simulink model "Studio7b"  (R2017b)
settings: Solver=ode45  StartTime=0.  StopTime=60  MaxStep=0.05  RelTol=1e-8  AbsTol=1e-8  EnableMultiTasking=on
settings Model: ExtModeTrigMode=oneshot  ExtModeArmWhenConnect=off  Creator=LEVIENKL  LastModifiedBy=carlislt
settings DataIOCC: SaveFormat=Array  SignalLoggingSaveFormat=ModelDataLogs  SaveOutput=off  SaveTime=off  SignalLoggingName=sigsOut
settings OptimizationCC: BlockReduction=off  BooleanDataType=off  ExpressionDepthLimit=2147483647  InitFltsAndDblsToZero=on  LifeSpan=inf
settings DebuggingCC: SaveWithParameterizedLinksMsg=none  UnderspecifiedInitializationDetection=Classic  MergeDetectMultiDrivingBlocksExec=none  SignalResolutionControl=TryResolveAllWithWarning  MultiTaskDSMMsg=warning  MultiTaskCondExecSysMsg=none  FcnCallInpInsideContextMsg=warning  AllowSymbolicDim=off  StateNameClashWarn=warning  SFUnexpectedBacktrackingDiag=warning  SFNoUnconditionalDefaultTransitionDiag=warning  SFExecutionAtInitializationDiag=none
settings HardwareCC: ProdBitPerPointer=32  ProdBitPerSizeT=32  ProdBitPerPtrDiffT=32  ProdLargestAtomicFloat=None  ProdIntDivRoundTo=Undefined  ProdEndianess=Unspecified  ProdWordSize=32  ProdHWDeviceType=32-bit Generic  TargetUnknown=on
settings ModelReferenceCC: PropagateSignalLabelsOutOfModel=off
settings CodeAppCC: StateflowObjectComments=on
settings GRTTargetCC: TargetFcnLib=ansi_tfl_tmw.mat  TargetLangStandard=C89/C90 (ANSI)  GeneratePreprocessorConditionals=Disable all  CombineOutputUpdateFcns=off  GRTInterface=on
settings ConfigComp: CovMetricSettings=dw  CovHtmlReporting=on  CovSaveCumulativeToWorkspaceVar=on  CovSaveSingleToWorkspaceVar=on  CovExternalEMLEnable=off  CovSFcnEnable=off

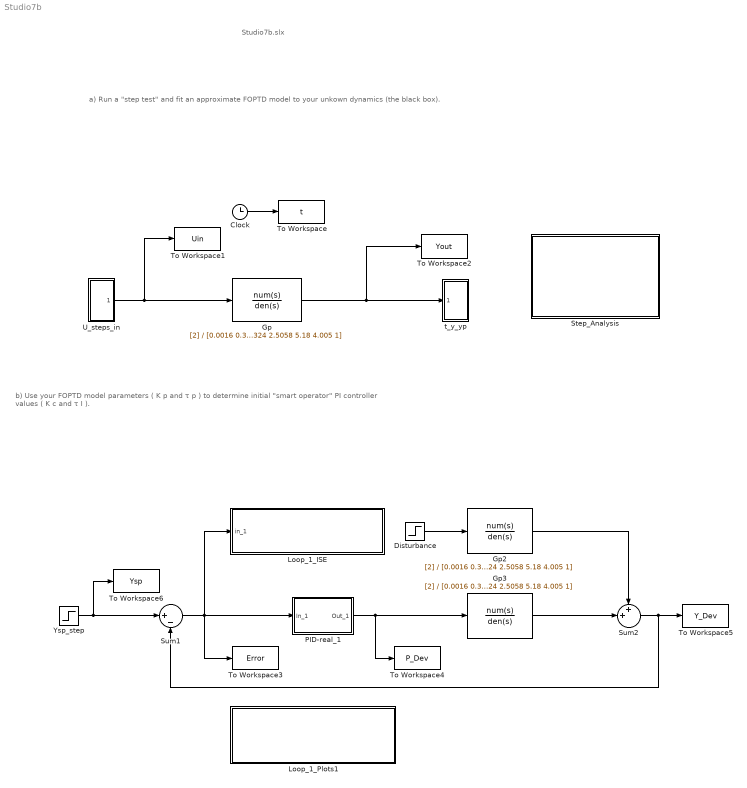
== system Studio7b ==
  note: Studio7b.slx
  note: a) Run a "step test" and fit an approximate FOPTD model to your unkown dynamics (the black box).
  note: b) Use your FOPTD model parameters ( K p and τ p ) to determine initial "smart operator" PI controller values ( K c and τ I ).
  Clock : Clock
  Disturbance : Step  Time=5  After=0  SampleTime=0
      settings: AttributesFormatString=%<Before> to %<After>\nat %<Time>
  Gp : TransferFcn  Numerator=[2]  Denominator=[0.0016 0.3324 2.5058 5.18 4.005 1]
  Gp2 : TransferFcn  Numerator=[2]  Denominator=[0.0016 0.3324 2.5058 5.18 4.005 1]
  Gp3 : TransferFcn  Numerator=[2]  Denominator=[0.0016 0.3324 2.5058 5.18 4.005 1]
  Loop_1_ISE : Subsystem  mask(Integral Squarred Evaluation - Loop 1){}
      settings: OpenFcn=ISE1
      mask Help: This block calculates and plots loop #1 ISE.
      mask Display: disp('After Loop 1 Simulation:\n Double Click for ISE evaluation\n (uses ISE1.p)')
  Loop_1_Plots1 : Subsystem  mask(Y,U,E Plots - Loop 1){}
      settings: OpenFcn=YPEplots
      mask Help: This block loop #1 Y,U,Error in 3x1 Figure Window.
      mask Display: disp('After Loop 1 Simulation:\n Double Click for Y, P, Error Plots\n (uses YPEplots.p)')
  PID-real_1 : Subsystem  mask(PID(with alpha) Controller for ChE 461){Kc=0.1, tauIi=1/10, tauD=0, alpha=0.05}
      mask prompts: Kc "Controller gain:"; tauIi "Inv of Integral time constant (careful - this is I action ! ) :"; tauD "Derivative time constant:"; alpha "Alpha value (small)::"
      mask help:
      | Enter expressions for controller gain,
      | inverse of integral time constant
      | and derivative time constant and alpha.
      settings: AttributesFormatString=Kc = %<Kc>\n1/TauI = %<tauIi>\nTauD = %<tauD>
      mask Help: This block implements a PID controller where parameters are entered for the Controller Gain, inverse of Integral time constant and Derivative time constant.  Alpha here is equal to 0.01.   Unmask this block to see how it works. The derivative term is implemented using a true derivative block.
      mask Display: disp('PIDalpha')
  Step_Analysis : Subsystem  mask(ASCII Datafile){}
      settings: OpenFcn=save tuin.dat tUin -ascii; save tyout.dat tYout -ascii; step2g
      mask Help: This block runs step2g\nin the MATLAB Command Window\nwith latest yout.dat data file.
      mask Display: disp('DOUBLE Click to\nRUN step2g\n\nGO TO Command Window !!')
  Sum1 : Sum  Inputs=|+-  SaturateOnIntegerOverflow=on  InputSameDT=on  OutDataTypeStr=Inherit: Same as first input
  Sum2 : Sum  Inputs=++|  SaturateOnIntegerOverflow=on  InputSameDT=on  OutDataTypeStr=Inherit: Same as first input
  To Workspace : ToWorkspace  VariableName=t  SampleTime=-1
  To Workspace1 : ToWorkspace  VariableName=Uin  SampleTime=-1
  To Workspace2 : ToWorkspace  VariableName=Yout  SampleTime=-1
  To Workspace3 : ToWorkspace  VariableName=Error  SampleTime=-1
  To Workspace4 : ToWorkspace  VariableName=P_Dev  SampleTime=-1
  To Workspace5 : ToWorkspace  VariableName=Y_Dev  SampleTime=-1
  To Workspace6 : ToWorkspace  VariableName=Ysp  SampleTime=-1
  U_steps_in : Subsystem
  Ysp_step : Step  Time=5  SampleTime=0
      settings: AttributesFormatString=%<Before> to %<After>\nat %<Time>
  t_y_yp : Subsystem
  wires:
  U_steps_in/1(out_1) -> To Workspace1/1, Gp/1
  Clock/1 -> To Workspace/1
  Gp/1 -> To Workspace2/1, t_y_yp/1(in_1)
  Disturbance/1 -> Gp2/1
  Gp3/1 -> Sum2/2
  PID-real_1/1(Out_1) -> Gp3/1, To Workspace4/1
  Gp2/1 -> Sum2/1
  Sum2/1 -> Sum1/2, To Workspace5/1
  Ysp_step/1 -> Sum1/1, To Workspace6/1
  Sum1/1 -> To Workspace3/1, Loop_1_ISE/1(in_1), PID-real_1/1(In_1)

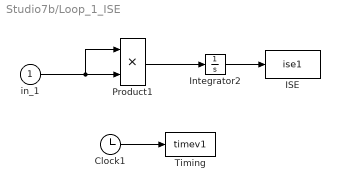
== system Studio7b/Loop_1_ISE ==
  in_1 : Inport
  Clock1 : Clock
  ISE : ToWorkspace  VariableName=ise1
      settings: MaxDataPoints=20000
  Integrator2 : Integrator
  Product1 : Product  SaturateOnIntegerOverflow=on  RndMeth=Zero  InputSameDT=on  OutDataTypeStr=Inherit: Same as first input
  Timing : ToWorkspace  VariableName=timev1
      settings: MaxDataPoints=20000
  wires:
  in_1/1 -> Product1/2, Product1/1
  Integrator2/1 -> ISE/1
  Clock1/1 -> Timing/1
  Product1/1 -> Integrator2/1

== system Studio7b/Loop_1_Plots1 ==

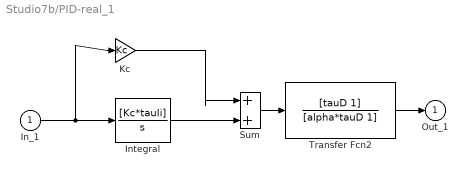
== system Studio7b/PID-real_1 ==
  In_1 : Inport
  Integral : TransferFcn  Numerator=[Kc*tauIi]  Denominator=[1 0]
  Kc : Gain  Gain=Kc  SaturateOnIntegerOverflow=on  OutDataTypeStr=Inherit: Same as input  ParamDataTypeStr=Inherit: Same as input
  Sum : Sum  SaturateOnIntegerOverflow=on  InputSameDT=on  OutDataTypeStr=Inherit: Same as first input
  Transfer Fcn2 : TransferFcn  Numerator=[tauD 1]  Denominator=[alpha*tauD 1]
  Out_1 : Outport
  wires:
  Transfer Fcn2/1 -> Out_1/1
  Sum/1 -> Transfer Fcn2/1
  In_1/1 -> Integral/1, Kc/1
  Integral/1 -> Sum/2
  Kc/1 -> Sum/1

== system Studio7b/Step_Analysis ==

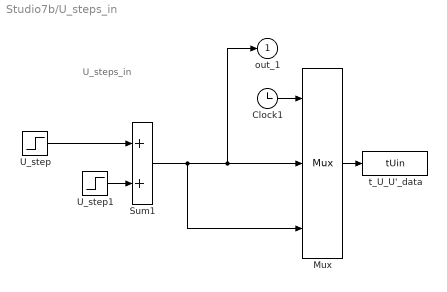
== system Studio7b/U_steps_in ==
  note: U_steps_in
  Clock1 : Clock
  Mux : Mux  Inputs=3
  Sum1 : Sum  SaturateOnIntegerOverflow=on  InputSameDT=on  OutDataTypeStr=Inherit: Same as first input
  U_step : Step  Time=0  After=0  SampleTime=0  ZeroCross=off
      settings: AttributesFormatString=%<Before> to %<After>\nat %<Time>
  U_step1 : Step  Time=0  After=0  SampleTime=0  ZeroCross=off
      settings: AttributesFormatString=%<Before> to %<After>\nat %<Time>
  t_U_U'_data : ToWorkspace  VariableName=tUin
      settings: MaxDataPoints=3000
  out_1 : Outport
  wires:
  Clock1/1 -> Mux/1
  U_step/1 -> Sum1/1
  U_step1/1 -> Sum1/2
  Sum1/1 -> Mux/3, Mux/2, out_1/1
  Mux/1 -> t_U_U'_data/1

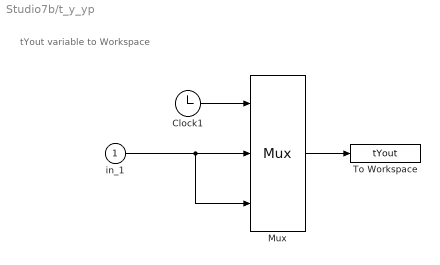
== system Studio7b/t_y_yp ==
  note: tYout variable
      | to Workspace
  in_1 : Inport
  Clock1 : Clock
  Mux : Mux  Inputs=3
  To Workspace : ToWorkspace  VariableName=tYout
      settings: MaxDataPoints=2000
  wires:
  Mux/1 -> To Workspace/1
  in_1/1 -> Mux/2, Mux/3
  Clock1/1 -> Mux/1
